simulink model "sampleModel1550"  (R2023a)
settings: Solver=VariableStepAuto  StartTime=0.0  StopTime=10.0  RelTol=1e-3
libraries: hdlsllib x5, simulink x2
settings Model: Creator=user1  LastModifiedBy=user1

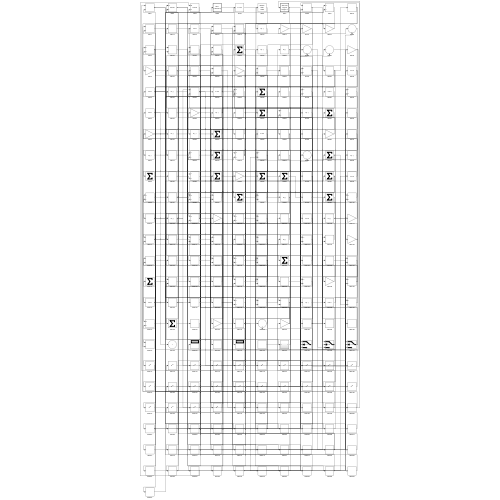
[thumbnail: Simulink's stored preview of the top-level diagram]
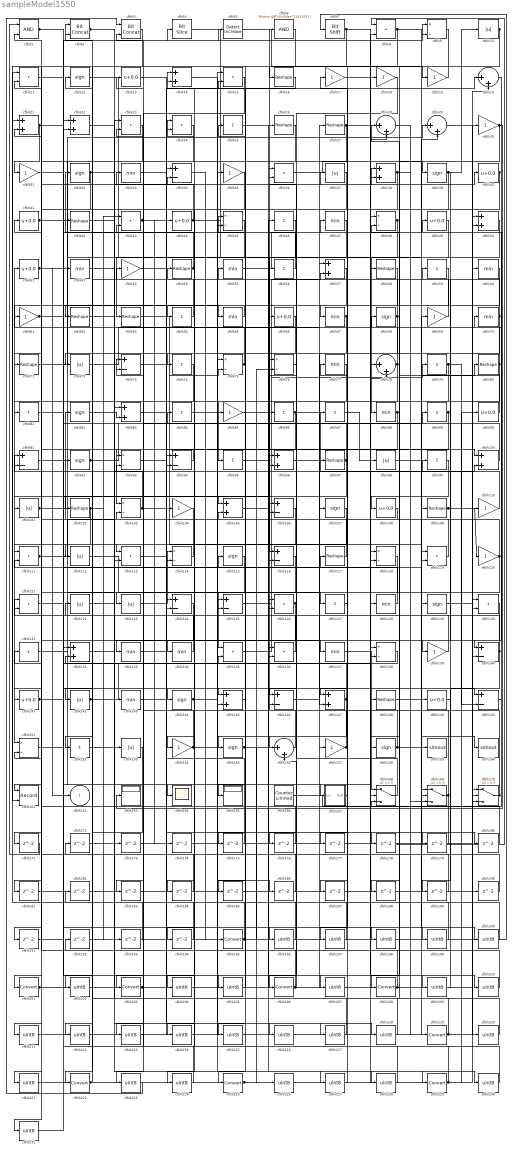
== system sampleModel1550 ==
  cfblk1 : Logic  AllPortsSameDT=off  OutDataTypeStr=boolean
  cfblk{10,37,72,98,101,112,122..123,142,153} (10 alike) : Abs  SaturateOnIntegerOverflow=off
  cfblk{14,21..22,38,50,57,83,96,100,105,132,145,147} (13 alike) : Sum
  cfblk{16,26..27,42,54,58,62..63,71,80,97,102,109,117,148} (15 alike) : Reshape
  cfblk{9,45,48,75..76,93,103,114,118,138,151} (11 alike) : Product  Inputs=*/  RndMeth=Zero  SaturateOnIntegerOverflow=on
  cfblk{17..19,30..31,35,53,61,69,85,104,110,120,139,154,157} (16 alike) : Gain
  cfblk{34,73,91,94,106,116,124..125,140,146,150} (11 alike) : Sum  Inputs=+-
  cfblk{12,32,39,68,82,92,107,115,129,144,155,158} (12 alike) : Signum
  cfblk{13,40..41,44,49,51,66,90,108,141,149} (11 alike) : Bias  Bias=0.0  SaturateOnIntegerOverflow=off
  cfblk{8,11,15,23..24,36,43,111,113,119,121,126,130,135..136} (15 alike) : DotProduct  OutDataTypeStr=Inherit: Inherit via internal rule
  cfblk{25,46,56,59,64,74,79,81,84,86..87,89,95,99,127,131,152} (17 alike) : Sum  Inputs=+
  cfblk{33,47,52,55,60,65,67,70,77,88,128,133..134,137,143} (15 alike) : MinMax
  cfblk{20,28..29,78,156} (5 alike) : Sum  Inputs=|++
  cfblk159 : ToWorkspace  VariableName=simout  SaveFormat=Timeseries  SampleTime=-1
  cfblk160 : ToWorkspace  VariableName=simout  SaveFormat=Timeseries  SampleTime=-1
  cfblk161 : Record  FileSettingsInternal="{\"entries\":[{\"content\":{\"excelSettings\":{\"content\":{},\"type\":\"Streamout.ExcelSettings\"}},\"type\":\"Streamout.FileSettingStorage\",\"uuid\":\"\"}],\"packageUris\":[\"http:\\/\\/schema.mathworks.com\\/mf0\\/streamout_blocks\\/R2020a\"],\"version\":\"1.0\"}"  Layout=[1 1]  SignalsInternal="{\"entries\":[{\"content\":{\"signals\":[{\"content\":{\"blockPath\":[],\"dimensions\":[1],\"domain\":\"\",\"lineColor\":\"#a2142f\",\"plots\":[1],\"port\":1,\"signalID\":1637,\"signalName\":\"XY Graph:1\"},\"type\":\"RecordBlkView.Signal\",\"uuid\":\"\"},{\"content\":{\"blockPath\":[],\"dimensions\":[1],\"domain\":\"\",\"lineColor\":\"#139fff\",\"plots\":[1],\"port\":2,\"signalID\":1640,\"signalName\":\"XY Graph:2\"},\"type\":\"RecordBlkView.Signal\",\"uuid\":\"\"}]},\"type\":\"RecordBlkView.InputSignals\",\"uuid\":\"\"}],\"packageUris\":[\"http:\\/\\/schema.mathworks.com\\/mf0\\/streamout_blocks\\/R2020a\"],\"version\":\"1.0\"}"  VisualizationBindings="{\"xyplotplugin\":{\"info\":[{\"series\":[{\"bindingParametersList\":[{\"parameter\":\"X-Axis\",\"signalID\":1637,\"signalName\":\"XY Graph:1\"},{\"parameter\":\"Y-Axis\",\"signalID\":1640,\"signalName\":\"XY Graph:2\"}],\"seriesID\":50005}],\"subplotID\":1}]}}"  CompatibilityTag=XY  st=-1
  cfblk163 : Display
  cfblk164 : Scope
  cfblk165 : Display
  cfblk166 : hdlsllib/Sources/Counter Limited  uplimit=7  tsamp=-1
  cfblk167 : Subsystem
      settings: LibrarySourceBlock=|
      | hdlsllib/Ports &
      | Subsystems/Subsystem
  cfblk168 : Switch  SaturateOnIntegerOverflow=off  InputSameDT=off
  cfblk169 : Switch  SaturateOnIntegerOverflow=off  InputSameDT=off
  cfblk170 : Switch  SaturateOnIntegerOverflow=off  InputSameDT=off
  cfblk{171..194} (24 alike) : Delay  SampleTime=1
  cfblk{195,201,203,206,208,219,222,225,229} (9 alike) : DataTypeConversion  SaturateOnIntegerOverflow=off  RndMeth=Floor
  cfblk{196..200,202,204..205,207,209..218,220..221,223..224,226..228,230..231} (28 alike) : DataTypeConversion  OutDataTypeStr=uint8  SaturateOnIntegerOverflow=off  RndMeth=Floor
  cfblk2 : hdlsllib/Logic and Bit Operations/Bit Concat  numInputs=2
  cfblk3 : hdlsllib/Logic and Bit Operations/Bit Concat  numInputs=2
  cfblk4 : hdlsllib/Logic and Bit Operations/Bit Slice  lidx=7  ridx=0
  cfblk5 : simulink/Logic and Bit Operations/Detect Increase  vinit=0.0  OutDataTypeStr=boolean
      settings: LibrarySourceBlock=|
      | hdlsllib/Logic and Bit
      | Operations/Detect
      | Increase
  cfblk6 : simulink/Logic and Bit Operations/Bitwise Operator  logicop=AND  UseBitMask=on  BitMask=bin2dec('11011001')  BitMaskRealWorld=Stored Integer
      settings: LibrarySourceBlock=|
      | hdlsllib/Logic and Bit
      | Operations/Bitwise
      | Operator
  cfblk7 : hdlsllib/Logic and Bit Operations/Bit Shift  mode=Shift Left Logical  N=0
  cfblk162 : Outport  VectorParamsAs1DForOutWhenUnconnected=off
  wires:
  cfblk48/1 -> cfblk63/1, cfblk67/1
  cfblk87/1 -> cfblk98/1
  cfblk102/1 -> cfblk43/1, cfblk173/1, cfblk231/1
  cfblk86/1 -> cfblk133/1, cfblk40/1
  cfblk5/1 -> cfblk19/1
  cfblk168/1 -> cfblk55/1
  cfblk95/1 -> cfblk79/1
  cfblk89/1 -> cfblk103/1, cfblk197/1
  cfblk90/1 -> cfblk54/1
  cfblk115/1 -> cfblk135/1
  cfblk140/1 -> cfblk48/2, cfblk2/2, cfblk189/1
  cfblk23/1 -> cfblk164/1
  cfblk166/1 -> cfblk49/1
  cfblk3/1 -> cfblk222/1
  cfblk120/1 -> cfblk82/1, cfblk126/2
  cfblk73/1 -> cfblk75/2
  cfblk30/1 -> cfblk163/1, cfblk188/1
  cfblk108/1 -> cfblk103/2
  cfblk109/1 -> cfblk120/1, cfblk150/2
  cfblk101/1 -> cfblk153/1, cfblk146/2
  cfblk99/1 -> cfblk208/1
  cfblk66/1 -> cfblk102/1
  cfblk158/1 -> cfblk53/1, cfblk80/1, cfblk200/1
  cfblk135/1 -> cfblk57/2
  cfblk56/1 -> cfblk6/1
  cfblk150/1 -> cfblk70/1
  cfblk80/1 -> cfblk51/1, cfblk106/2
  cfblk34/1 -> cfblk195/1
  cfblk59/1 -> cfblk151/1
  cfblk155/1 -> cfblk226/1, cfblk228/1
  cfblk170/1 -> cfblk26/1, cfblk126/1
  cfblk25/1 -> cfblk137/1
  cfblk32/1 -> cfblk81/1, cfblk167/1(In1)
  cfblk123/1 -> cfblk114/1
  cfblk35/1 -> cfblk201/1
  cfblk71/1 -> cfblk47/1
  cfblk77/1 -> cfblk95/1
  cfblk7/1 -> cfblk118/1, cfblk161/2
  cfblk51/1 -> cfblk29/1, cfblk162/1
  cfblk44/1 -> cfblk88/1, cfblk21/2
  cfblk65/1 -> cfblk62/1
  cfblk63/1 -> cfblk149/1
  cfblk98/1 -> cfblk169/1
  cfblk147/1 -> cfblk45/2, cfblk175/1, cfblk176/1
  cfblk72/1 -> cfblk27/1
  cfblk169/1 -> cfblk68/1, cfblk168/3
  cfblk148/1 -> cfblk109/1
  cfblk167/1(Out1) -> cfblk77/1
  cfblk46/1 -> cfblk116/1
  cfblk43/1 -> cfblk20/1, cfblk174/1
  cfblk36/1 -> cfblk39/1
  cfblk156/1 -> cfblk14/1
  cfblk12/1 -> cfblk124/1
  cfblk137/1 -> cfblk168/1
  cfblk146/1 -> cfblk107/1
  cfblk112/1 -> cfblk124/2
  cfblk70/1 -> cfblk123/1, cfblk36/2, cfblk114/2
  cfblk4/1 -> cfblk159/1
  cfblk111/1 -> cfblk83/1, cfblk168/2
  cfblk6/1 -> cfblk165/1
  cfblk142/1 -> cfblk78/1, cfblk193/1
  cfblk19/1 -> cfblk16/1
  cfblk132/1 -> cfblk37/1
  cfblk92/1 -> cfblk44/1, cfblk100/2
  cfblk110/1 -> cfblk17/1
  cfblk61/1 -> cfblk65/1, cfblk9/2
  cfblk22/1 -> cfblk229/1
  cfblk127/1 -> cfblk147/1
  cfblk157/1 -> cfblk66/1, cfblk93/2
  cfblk151/1 -> cfblk52/1
  cfblk68/1 -> cfblk36/1, cfblk187/1
  cfblk9/1 -> cfblk125/1
  cfblk67/1 -> cfblk147/2, cfblk156/1
  cfblk39/1 -> cfblk10/1, cfblk111/1, cfblk113/2, cfblk139/1
  cfblk143/1 -> cfblk94/2
  cfblk118/1 -> cfblk134/1
  cfblk60/1 -> cfblk225/1
  cfblk134/1 -> cfblk121/1
  cfblk8/1 -> cfblk101/1, cfblk160/1
  cfblk149/1 -> cfblk59/1
  cfblk82/1 -> cfblk83/2
  cfblk27/1 -> cfblk9/1, cfblk181/1
  cfblk55/1 -> cfblk29/2
  cfblk83/1 -> cfblk138/1
  cfblk76/1 -> cfblk146/1
  cfblk105/1 -> cfblk116/2
  cfblk96/1 -> cfblk87/1
  cfblk16/1 -> cfblk14/2
  cfblk93/1 -> cfblk127/1
  cfblk139/1 -> cfblk25/1
  cfblk106/1 -> cfblk113/1
  cfblk28/1 -> cfblk219/1
  cfblk97/1 -> cfblk76/1, cfblk145/2, cfblk221/1
  cfblk94/1 -> cfblk93/1
  cfblk144/1 -> cfblk179/1, cfblk180/1
  cfblk131/1 -> cfblk148/1
  cfblk154/1 -> cfblk73/2, cfblk218/1
  cfblk107/1 -> cfblk125/2
  cfblk62/1 -> cfblk136/2
  cfblk57/1 -> cfblk154/1
  cfblk122/1 -> cfblk38/1
  cfblk38/1 -> cfblk96/2, cfblk169/3
  cfblk21/1 -> cfblk31/1, cfblk4/1, cfblk71/1
  cfblk41/1 -> cfblk138/2, cfblk5/1, cfblk207/1
  cfblk42/1 -> cfblk143/1
  cfblk13/1 -> cfblk100/1
  cfblk15/1 -> cfblk203/1
  cfblk1/1 -> cfblk92/1, cfblk145/1
  cfblk75/1 -> cfblk74/1, cfblk61/1
  cfblk64/1 -> cfblk13/1
  cfblk40/1 -> cfblk152/1, cfblk64/1
  cfblk20/1 -> cfblk140/1
  cfblk31/1 -> cfblk132/1
  cfblk69/1 -> cfblk2/1
  cfblk24/1 -> cfblk142/1
  cfblk79/1 -> cfblk110/1, cfblk224/1
  cfblk91/1 -> cfblk105/1
  cfblk121/1 -> cfblk117/1
  cfblk103/1 -> cfblk91/1, cfblk150/1
  cfblk125/1 -> cfblk69/1
  cfblk81/1 -> cfblk45/1
  cfblk49/1 -> cfblk86/1
  cfblk29/1 -> cfblk170/1
  cfblk54/1 -> cfblk32/1, cfblk12/1
  cfblk37/1 -> cfblk72/1
  cfblk114/1 -> cfblk112/1
  cfblk138/1 -> cfblk132/2
  cfblk18/1 -> cfblk206/1
  cfblk126/1 -> cfblk184/1, cfblk185/1
  cfblk117/1 -> cfblk41/1
  cfblk141/1 -> cfblk135/2, cfblk89/1
  cfblk136/1 -> cfblk24/1
  cfblk119/1 -> cfblk42/1
  cfblk128/1 -> cfblk91/2
  cfblk10/1 -> cfblk158/1, cfblk177/1
  cfblk78/1 -> cfblk56/1, cfblk161/1, cfblk155/1
  cfblk100/1 -> cfblk73/1
  cfblk2/1 -> cfblk106/1, cfblk144/1
  cfblk88/1 -> cfblk141/1, cfblk108/1
  cfblk74/1 -> cfblk171/1
  cfblk171/1 -> cfblk1/1
  cfblk172/1 -> cfblk130/1
  cfblk173/1 -> cfblk75/1
  cfblk174/1 -> cfblk136/1
  cfblk175/1 -> cfblk94/1
  cfblk176/1 -> cfblk24/2
  cfblk177/1 -> cfblk140/2
  cfblk113/1 -> cfblk178/1
  cfblk178/1 -> cfblk8/1
  cfblk179/1 -> cfblk169/2
  cfblk180/1 -> cfblk121/2
  cfblk181/1 -> cfblk118/2
  cfblk182/1 -> cfblk119/2
  cfblk26/1 -> cfblk183/1
  cfblk183/1 -> cfblk48/1
  cfblk184/1 -> cfblk151/2
  cfblk185/1 -> cfblk170/3
  cfblk14/1 -> cfblk186/1
  cfblk186/1 -> cfblk96/1
  cfblk187/1 -> cfblk38/2
  cfblk188/1 -> cfblk20/2
  cfblk189/1 -> cfblk43/2
  cfblk190/1 -> cfblk57/1
  cfblk124/1 -> cfblk191/1
  cfblk192/1 -> cfblk78/2
  cfblk193/1 -> cfblk1/2
  cfblk47/1 -> cfblk194/1
  cfblk194/1 -> cfblk21/1
  cfblk195/1 -> cfblk131/1, cfblk76/2, cfblk115/1
  cfblk133/1 -> cfblk196/1
  cfblk196/1 -> cfblk34/1
  cfblk197/1 -> cfblk34/2
  cfblk11/1 -> cfblk198/1
  cfblk198/1 -> cfblk7/1
  cfblk53/1 -> cfblk199/1
  cfblk199/1 -> cfblk11/1
  cfblk200/1 -> cfblk11/2
  cfblk201/1 -> cfblk157/1, cfblk46/1
  cfblk153/1 -> cfblk202/1
  cfblk202/1 -> cfblk35/1
  cfblk203/1 -> cfblk128/1, cfblk8/2
  cfblk130/1 -> cfblk204/1
  cfblk204/1 -> cfblk15/1
  cfblk191/1 -> cfblk205/1
  cfblk205/1 -> cfblk15/2
  cfblk206/1 -> cfblk156/2, cfblk111/2, cfblk129/1
  cfblk207/1 -> cfblk18/1
  cfblk208/1 -> cfblk190/1, cfblk105/2
  cfblk17/1 -> cfblk209/1
  cfblk209/1 -> cfblk99/1
  cfblk85/1 -> cfblk210/1
  cfblk210/1 -> cfblk172/1
  cfblk116/1 -> cfblk211/1
  cfblk211/1 -> cfblk85/1
  cfblk104/1 -> cfblk212/1
  cfblk212/1 -> cfblk130/2
  cfblk58/1 -> cfblk213/1
  cfblk213/1 -> cfblk104/1
  cfblk50/1 -> cfblk214/1
  cfblk214/1 -> cfblk119/1
  cfblk145/1 -> cfblk215/1
  cfblk215/1 -> cfblk50/1
  cfblk52/1 -> cfblk216/1
  cfblk216/1 -> cfblk50/2
  cfblk33/1 -> cfblk217/1
  cfblk217/1 -> cfblk23/1
  cfblk218/1 -> cfblk33/1
  cfblk219/1 -> cfblk182/1, cfblk23/2
  cfblk129/1 -> cfblk220/1
  cfblk220/1 -> cfblk28/1
  cfblk221/1 -> cfblk28/2
  cfblk222/1 -> cfblk30/1, cfblk122/1
  cfblk45/1 -> cfblk223/1
  cfblk223/1 -> cfblk3/1
  cfblk224/1 -> cfblk3/2
  cfblk225/1 -> cfblk170/2, cfblk58/1
  cfblk226/1 -> cfblk60/1
  cfblk84/1 -> cfblk227/1
  cfblk227/1 -> cfblk97/1
  cfblk228/1 -> cfblk84/1
  cfblk229/1 -> cfblk192/1, cfblk90/1
  cfblk152/1 -> cfblk230/1
  cfblk230/1 -> cfblk22/1
  cfblk231/1 -> cfblk22/2

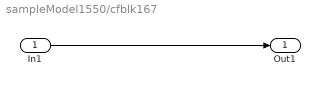
== system sampleModel1550/cfblk167 ==
  In1 : Inport
  Out1 : Outport
  wires:
  In1/1 -> Out1/1
